simulink model "simulink_with_rectify"  (R2020a)
settings: Solver=ode45  StartTime=0.0  StopTime=10.0  RelTol=1e-3
settings Model: Creator=oyh  LastModifiedBy=oyh

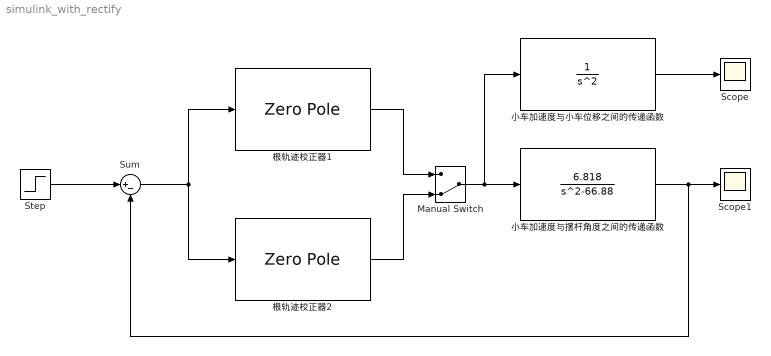
== system simulink_with_rectify ==
  Manual Switch : ManualSwitch  CurrentSetting=0
  Scope : Scope
  Scope1 : Scope
  Step : Step  Time=0  After=0.1  SampleTime=0
  Sum : Sum  Inputs=|+-
  小车加速度与小车位移之间的传递函数 : TransferFcn  Denominator=[1 0 0]
  小车加速度与摆杆角度之间的传递函数 : TransferFcn  Numerator=[6.818]  Denominator=[1 0 -66.88]
  根轨迹校正器1 : ZeroPole  Zeros=[-7.876]  Poles=[-23.25]  Gain=[53.687]
  根轨迹校正器2 : ZeroPole  Zeros=[-26.39]  Poles=[-52.24]  Gain=[297.07]
  wires:
  Step/1 -> Sum/1
  Sum/1 -> 根轨迹校正器2/1, 根轨迹校正器1/1
  根轨迹校正器1/1 -> Manual Switch/1
  根轨迹校正器2/1 -> Manual Switch/2
  Manual Switch/1 -> 小车加速度与小车位移之间的传递函数/1, 小车加速度与摆杆角度之间的传递函数/1
  小车加速度与小车位移之间的传递函数/1 -> Scope/1
  小车加速度与摆杆角度之间的传递函数/1 -> Sum/2, Scope1/1
